simulink model "PianoToSineModel"  (R2018b)
settings: Solver=VariableStepAuto  StartTime=0.0  StopTime=10.0  RelTol=1e-3
libraries: dspsrcs4 x1
settings Model: Creator=asus  LastModifiedBy=asus

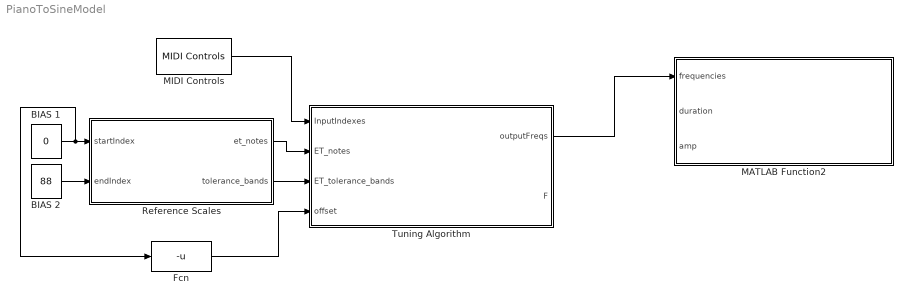
== system PianoToSineModel ==
  BIAS 1 : Constant  Value=0
  BIAS 2 : Constant  Value=88
  Fcn : Fcn  Expr=-u
  MATLAB Function2 : MATLAB Function  TreatAsAtomicUnit=on
  MIDI Controls : dspsrcs4/MIDI Controls  UseSpecifiedDevice=Default  DeviceName=''  UseSpecifiedControls=Respond to any control  ControlNumbers=0  InitialValues=0  SyncAtStart=off  RawUint8=Raw MIDI (0 - 127)
      settings: SourceProductName=DSP System Toolbox  SourceProductBaseCode=DS
  Reference Scales : MATLAB Function  TreatAsAtomicUnit=on
  "Tuning Algorithm " : MATLAB Function  TreatAsAtomicUnit=on
  wires:
  Fcn/1 -> "Tuning Algorithm "/4(offset)
  Reference Scales/2(tolerance_bands) -> "Tuning Algorithm "/3(ET_tolerance_bands)
  Reference Scales/1(et_notes) -> "Tuning Algorithm "/2(ET_notes)
  MIDI Controls/1 -> "Tuning Algorithm "/1(InputIndexes)
  BIAS 2/1 -> Reference Scales/2(endIndex)
  BIAS 1/1 -> Fcn/1, Reference Scales/1(startIndex)
  "Tuning Algorithm "/1(outputFreqs) -> MATLAB Function2/1(frequencies)

== matlab function PianoToSineModel/Reference Scales ==
  data: startIndex input; et_notes output; endIndex input; tolerance_bands output
function [et_notes, tolerance_bands] = generateETNotes(startIndex, endIndex)
%GENERATEETNOTES returns array [startIndex, endIndex] of equal
% temperament frequencies.  Assumes A4=440.

A4 = 440;         % frequency typically associated with A4 in western music
A4_pos = 49;      % A4 is 49th note on piano
max_cent_change = 49;   % controls algo's wiggle room
index = 1;

et_notes = ones(1, endIndex-startIndex+1);
for i=startIndex:endIndex
    et_notes(index) = A4*(2^(1/12))^(i-A4_pos);
    index = index+1;
end

tolerance_bands = zeros(2,endIndex-startIndex+1);
for i = 1:(endIndex-startIndex+1)
    tolerance_bands(1,i) = changeByCents(et_notes(i), -1*max_cent_change);
    tolerance_bands(2,i) = changeByCents(et_notes(i), max_cent_change);
end
end

function [outputFreq] = changeByCents(startingFreq, deltCents)
    outputFreq = startingFreq * 2^(deltCents/1200);
end

== matlab function PianoToSineModel/Tuning Algorithm  ==
  data: InputIndexes input; outputFreqs output; ET_notes input; ET_tolerance_bands input; offset input; F output
function [outputFreqs, F] = Algorithm1(InputIndexes, ET_notes, ET_tolerance_bands, offset)
%ALGORITHM1 Seeks to maximize the fundamental Frequency st. adjusting the
%original notes as little as possible
tic  % start timer

%adjustable params:
max_multiple = 24;

num_notes = length(InputIndexes);
adj_distances = zeros(1, num_notes);
for i = 1:(num_notes - 1)
    adj_distances(i) = ET_notes(InputIndexes(i+1)) - ET_notes(InputIndexes(i));
end
adj_distances(num_notes) = ET_notes(InputIndexes(1));

starting_F = min(adj_distances);

%Search by iterating down the OT series starting from starting_F
Findex = find(ET_notes > starting_F, 1);

while 1
    if Findex == 0
        outputFreqs = [];  % if doesn't work should probably just play original freqs
        break
    end
    F = ET_notes(Findex);
    max_overtones = min(ET_tolerance_bands(2,num_notes), max_multiple);
    multipleF = F.*(1:max_overtones);
    ovt = 1;
    outputFreqs = zeros(1,num_notes);
    
    for note = 1:num_notes
        index = InputIndexes(note);
        low_bound = ET_tolerance_bands(1,index-offset);
        up_bound = ET_tolerance_bands(2,index-offset);
        while ovt <= max_overtones
           corrected_freq = multipleF(ovt);
           ovt = ovt+1;
           if corrected_freq >= low_bound && corrected_freq <= up_bound
               outputFreqs(note) = corrected_freq;
               break;
           end
        end
    end
    if outputFreqs(num_notes) == 0
        outputFreqs = [];
        Findex = Findex - 1;
    else
        break;
    end
end
toc  %end timer


end

== matlab function PianoToSineModel/MATLAB Function2 ==
  data: frequencies input; duration input; amp input
function playNotes(frequencies,duration, amp)
%PLAYNOTES Summary of this function goes here
%   Detailed explanation goes here

    %temporary fix: for some reason, the first note starts earlier than the
    %others, so fixing this by adding a leading 0
    frequencies = [0, frequencies];

    sampling_frequency = 8192;
    values = 0:(1/sampling_frequency):duration;
    test = 2*pi*frequencies'*values;
    a = amp*sin(test);
    for i=1:size(a,1)
        sound(a(i,:));
    end
end
